simulink subsystem "custom_maneuver"  (R2020a)
settings: Solver=VariableStepAuto  StartTime=0.0  StopTime=10.0  RelTol=1e-3
libraries: simulink x1
settings Model: Creator=Fil  LastModifiedBy=Fil

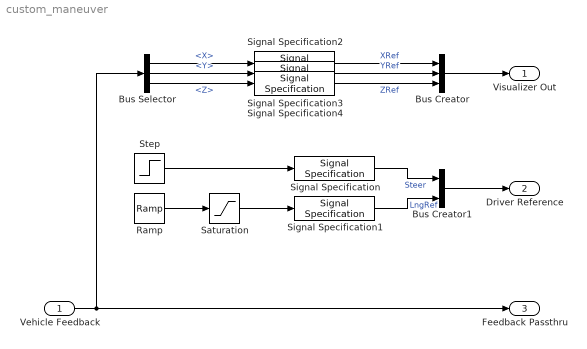
== system custom_maneuver ==
  Vehicle Feedback : Inport
  Bus Creator : BusCreator  Inputs=3
  Bus Creator1 : BusCreator  Inputs=2
  Bus Selector : BusSelector  OutputSignals=Body.X,Body.Y,Body.Z
  Ramp : simulink/Sources/Ramp  slope=5  start=0  InitialOutput=0
  Saturation : Saturate  UpperLimit=130  LowerLimit=50
  Signal Specification : SignalSpecification  Unit=deg
  Signal Specification1 : SignalSpecification  Unit=km/h
  Signal Specification2 : SignalSpecification
  Signal Specification3 : SignalSpecification
  Signal Specification4 : SignalSpecification
  Step : Step  Time=20  After=120  SampleTime=0
  Visualizer Out : Outport
  Driver Reference : Outport  Port=2
  Feedback Passthru : Outport  Port=3
  wires:
  Vehicle Feedback/1 -> Feedback Passthru/1, Bus Selector/1
  Bus Creator/1 -> Visualizer Out/1
  Bus Selector/1 -> Signal Specification2/1  "<X>"
  Bus Selector/2 -> Signal Specification3/1  "<Y>"
  Bus Selector/3 -> Signal Specification4/1  "<Z>"
  Bus Creator1/1 -> Driver Reference/1
  Signal Specification/1 -> Bus Creator1/1  "Steer"
  Signal Specification1/1 -> Bus Creator1/2  "LngRef"
  Step/1 -> Signal Specification/1
  Ramp/1 -> Saturation/1
  Saturation/1 -> Signal Specification1/1
  Signal Specification2/1 -> Bus Creator/1  "XRef"
  Signal Specification3/1 -> Bus Creator/2  "YRef"
  Signal Specification4/1 -> Bus Creator/3  "ZRef"
